simulink model "DCMG_SG"  (R2016a)
settings: Solver=FixedStepDiscrete  StartTime=0.0  StopTime=inf  FixedStep=.1  RelTol=1e-3
StartFcn:
  | h=add_exec_event_listener('GridSGHardware/GUIScope','PostOutputs',@GUIScope);
undefined symbols (not defined in the file or in its folder): Manual
libraries: opclib x4
settings Model: Creator=Don  LastModifiedBy=Microgrid_Project
settings DataIOCC: SaveFormat=Array  SignalLoggingSaveFormat=ModelDataLogs
settings OptimizationCC: ExpressionDepthLimit=2147483647
settings DebuggingCC: UnderspecifiedInitializationDetection=Classic  MergeDetectMultiDrivingBlocksExec=none  SolverPrmCheckMsg=warning  FcnCallInpInsideContextMsg=UseLocalSettings  StateNameClashWarn=warning
settings HardwareCC: ProdBitPerPointer=32  ProdLargestAtomicFloat=None  ProdIntDivRoundTo=Undefined  ProdEndianess=Unspecified  ProdWordSize=32  ProdHWDeviceType=32-bit Generic
settings ModelReferenceCC: PropagateSignalLabelsOutOfModel=off
settings GRTTargetCC: CombineOutputUpdateFcns=off  GRTInterface=on
settings ConfigComp: CovModelRefEnable=Off

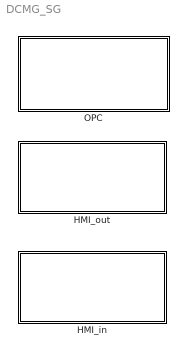
== system DCMG_SG ==
  HMI_in : Subsystem
  HMI_out : Subsystem
  OPC : Subsystem

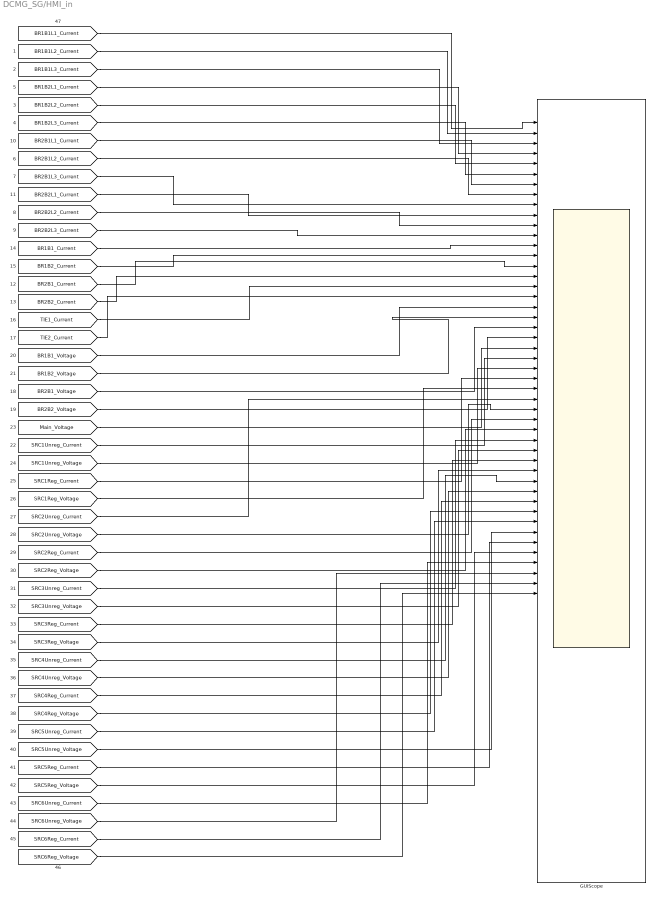
== system DCMG_SG/HMI_in ==
  GUIScope : Scope  NumInputPorts=73
  wires:
  [TIE2_Current] -> GUIScope/18
  [TIE1_Current] -> GUIScope/17
  [BR1B1_Voltage] -> GUIScope/19
  [BR2B2_Current] -> GUIScope/16
  [BR1B2_Voltage] -> GUIScope/20
  [BR2B1_Current] -> GUIScope/15
  [BR2B1_Voltage] -> GUIScope/21
  [BR1B2_Current] -> GUIScope/14
  [BR2B2_Voltage] -> GUIScope/22
  [BR1B1_Current] -> GUIScope/13
  [Main_Voltage] -> GUIScope/23
  [BR2B2L3_Current] -> GUIScope/12
  [SRC1Unreg_Current] -> GUIScope/24
  [BR2B2L2_Current] -> GUIScope/11
  [SRC1Unreg_Voltage] -> GUIScope/25
  [BR2B2L1_Current] -> GUIScope/10
  [SRC1Reg_Current] -> GUIScope/26
  [BR2B1L3_Current] -> GUIScope/9
  [SRC1Reg_Voltage] -> GUIScope/27
  [BR2B1L2_Current] -> GUIScope/8
  [SRC2Unreg_Current] -> GUIScope/28
  [BR2B1L1_Current] -> GUIScope/7
  [SRC2Unreg_Voltage] -> GUIScope/29
  [BR1B2L3_Current] -> GUIScope/6
  [SRC2Reg_Current] -> GUIScope/30
  [BR1B2L2_Current] -> GUIScope/5
  [SRC2Reg_Voltage] -> GUIScope/31
  [BR1B2L1_Current] -> GUIScope/4
  [SRC3Unreg_Current] -> GUIScope/32
  [BR1B1L3_Current] -> GUIScope/3
  [SRC3Unreg_Voltage] -> GUIScope/33
  [BR1B1L2_Current] -> GUIScope/2
  [SRC3Reg_Current] -> GUIScope/34
  [BR1B1L1_Current] -> GUIScope/1
  [SRC3Reg_Voltage] -> GUIScope/35
  [SRC4Unreg_Current] -> GUIScope/36
  [SRC4Unreg_Voltage] -> GUIScope/37
  [SRC4Reg_Current] -> GUIScope/38
  [SRC4Reg_Voltage] -> GUIScope/39
  [SRC5Unreg_Current] -> GUIScope/40
  [SRC5Unreg_Voltage] -> GUIScope/41
  [SRC5Reg_Current] -> GUIScope/42
  [SRC5Reg_Voltage] -> GUIScope/43
  [SRC6Unreg_Current] -> GUIScope/44
  [SRC6Unreg_Voltage] -> GUIScope/45
  [SRC6Reg_Current] -> GUIScope/46
  [SRC6Reg_Voltage] -> GUIScope/47

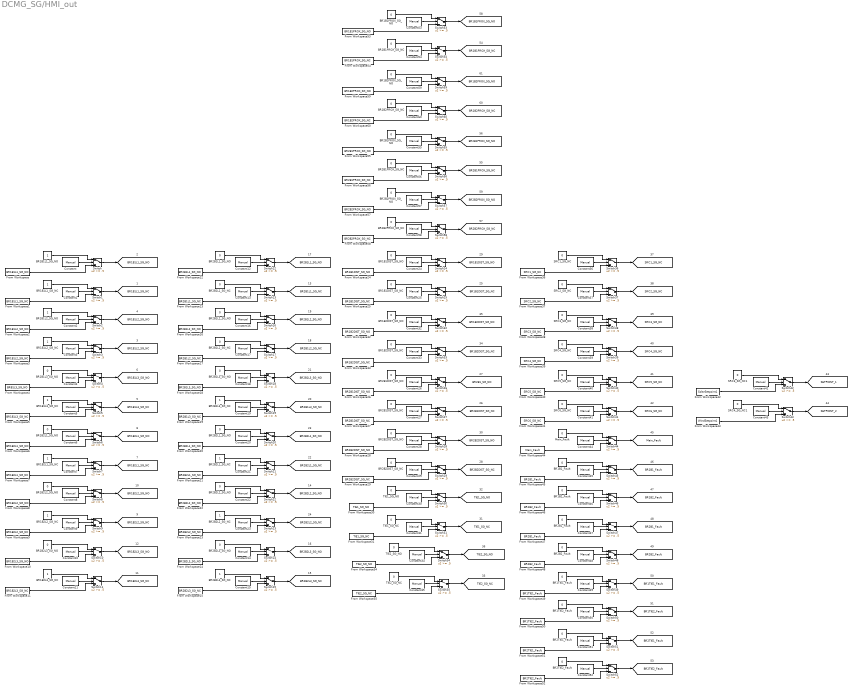
== system DCMG_SG/HMI_out ==
  BR1B1DIST_SG_NC : Constant  Value=0
  BR1B1DIST_SG_NO : Constant  Value=0
  BR1B1L1_SG_NC : Constant
  BR1B1L1_SG_NO : Constant
  BR1B1L2_SG_NC : Constant
  BR1B1L2_SG_NO : Constant
  BR1B1L3_SG_NC : Constant
  BR1B1L3_SG_NO : Constant  Value=0
  BR1B1PROX_SG_NC : Constant  Value=0
  BR1B1PROX_SG_NO : Constant  Value=0
  BR1B1_Fault : Constant  Value=0
  BR1B2DIST_SG_NC : Constant  Value=0
  BR1B2DIST_SG_NO : Constant  Value=0
  BR1B2L1_SG_NC : Constant
  BR1B2L1_SG_NO : Constant  Value=0
  BR1B2L2_SG_NC : Constant
  BR1B2L2_SG_NO : Constant  Value=0
  BR1B2L3_SG_NC : Constant
  BR1B2L3_SG_NO : Constant  Value=0
  BR1B2PROX_SG_NC : Constant  Value=0
  BR1B2PROX_SG_NO : Constant  Value=0
  BR1B2_Fault : Constant  Value=0
  BR1TIE1_Fault : Constant  Value=0
  BR1TIE2_Fault : Constant  Value=0
  BR2B1DIST_SG_NC : Constant  Value=0
  BR2B1DIST_SG_NO : Constant  Value=0
  BR2B1L1_SG_NC : Constant  Value=0
  BR2B1L1_SG_NO : Constant  Value=0
  BR2B1L2_SG_NC : Constant  Value=0
  BR2B1L2_SG_NO : Constant  Value=0
  BR2B1L3_SG_NC : Constant
  BR2B1L3_SG_NO : Constant  Value=0
  BR2B1PROX_SG_NC : Constant  Value=0
  BR2B1PROX_SG_NO : Constant  Value=0
  BR2B1_Fault : Constant  Value=0
  BR2B2DIST_SG_NC : Constant  Value=0
  BR2B2DIST_SG_NO : Constant  Value=0
  BR2B2L1_SG_NC : Constant
  BR2B2L1_SG_NO : Constant  Value=0
  BR2B2L2_SG_NC : Constant
  BR2B2L2_SG_NO : Constant  Value=0
  BR2B2L3_SG_NC : Constant
  BR2B2L3_SG_NO : Constant  Value=0
  BR2B2PROX_SG_NC : Constant  Value=0
  BR2B2PROX_SG_NO : Constant  Value=0
  BR2B2_Fault : Constant  Value=0
  BR2TIE1_Fault : Constant  Value=0
  BR2TIE2_Fault : Constant  Value=0
  Constant{,1..60} (61 alike) : Constant  Value=Manual
  From Workspace : FromWorkspace  VariableName=BR1B1L1_SG_NO  SampleTime=0  Interpolate=off  OutputAfterFinalValue=Holding final value
  From Workspace1 : FromWorkspace  VariableName=BR1B1L1_SG_NC  SampleTime=0  Interpolate=off  OutputAfterFinalValue=Holding final value
  From Workspace10 : FromWorkspace  VariableName=BR1B2L3_SG_NO  SampleTime=0  Interpolate=off  OutputAfterFinalValue=Holding final value
  From Workspace11 : FromWorkspace  VariableName=BR1B2L3_SG_NC  SampleTime=0  Interpolate=off  OutputAfterFinalValue=Holding final value
  From Workspace12 : FromWorkspace  VariableName=BR2B1L1_SG_NO  SampleTime=0  Interpolate=off  OutputAfterFinalValue=Holding final value
  From Workspace13 : FromWorkspace  VariableName=BR2B1L1_SG_NC  SampleTime=0  Interpolate=off  OutputAfterFinalValue=Holding final value
  From Workspace14 : FromWorkspace  VariableName=BR2B2L3_SG_NO  SampleTime=0  Interpolate=off  OutputAfterFinalValue=Holding final value
  From Workspace15 : FromWorkspace  VariableName=BR2B2L3_SG_NC  SampleTime=0  Interpolate=off  OutputAfterFinalValue=Holding final value
  From Workspace16 : FromWorkspace  VariableName=BR2B1L2_SG_NO  SampleTime=0  Interpolate=off  OutputAfterFinalValue=Holding final value
  From Workspace17 : FromWorkspace  VariableName=BR2B1L2_SG_NC  SampleTime=0  Interpolate=off  OutputAfterFinalValue=Holding final value
  From Workspace18 : FromWorkspace  VariableName=BR2B1L3_SG_NO  SampleTime=0  Interpolate=off  OutputAfterFinalValue=Holding final value
  From Workspace19 : FromWorkspace  VariableName=BR2B1L3_SG_NC  SampleTime=0  Interpolate=off  OutputAfterFinalValue=Holding final value
  From Workspace2 : FromWorkspace  VariableName=BR1B1L2_SG_NO  SampleTime=0  Interpolate=off  OutputAfterFinalValue=Holding final value
  From Workspace20 : FromWorkspace  VariableName=BR2B2L1_SG_NO  SampleTime=0  Interpolate=off  OutputAfterFinalValue=Holding final value
  From Workspace21 : FromWorkspace  VariableName=BR2B2L1_SG_NC  SampleTime=0  Interpolate=off  OutputAfterFinalValue=Holding final value
  From Workspace22 : FromWorkspace  VariableName=BR2B2L2_SG_NO  SampleTime=0  Interpolate=off  OutputAfterFinalValue=Holding final value
  From Workspace23 : FromWorkspace  VariableName=BR2B2L2_SG_NC  SampleTime=0  Interpolate=off  OutputAfterFinalValue=Holding final value
  From Workspace24 : FromWorkspace  VariableName=BR1B1DIST_SG_NO  SampleTime=0  Interpolate=off  OutputAfterFinalValue=Holding final value
  From Workspace25 : FromWorkspace  VariableName=BR1B1DIST_SG_NC  SampleTime=0  Interpolate=off  OutputAfterFinalValue=Holding final value
  From Workspace26 : FromWorkspace  VariableName=BR2B1DIST_SG_NO  SampleTime=0  Interpolate=off  OutputAfterFinalValue=Holding final value
  From Workspace27 : FromWorkspace  VariableName=BR2B1DIST_SG_NC  SampleTime=0  Interpolate=off  OutputAfterFinalValue=Holding final value
  From Workspace28 : FromWorkspace  VariableName=BR2B2DIST_SG_NO  SampleTime=0  Interpolate=off  OutputAfterFinalValue=Holding final value
  From Workspace29 : FromWorkspace  VariableName=BR2B2DIST_SG_NC  SampleTime=0  Interpolate=off  OutputAfterFinalValue=Holding final value
  From Workspace3 : FromWorkspace  VariableName=BR1B1L2_SG_NC  SampleTime=0  Interpolate=off  OutputAfterFinalValue=Holding final value
  From Workspace30 : FromWorkspace  VariableName=TIE1_SG_NO  SampleTime=0  Interpolate=off  OutputAfterFinalValue=Holding final value
  From Workspace31 : FromWorkspace  VariableName=TIE1_SG_NC  SampleTime=0  Interpolate=off  OutputAfterFinalValue=Holding final value
  From Workspace32 : FromWorkspace  VariableName=BR1B2DIST_SG_NO  SampleTime=0  Interpolate=off  OutputAfterFinalValue=Holding final value
  From Workspace33 : FromWorkspace  VariableName=BR1B2DIST_SG_NC  SampleTime=0  Interpolate=off  OutputAfterFinalValue=Holding final value
  From Workspace34 : FromWorkspace  VariableName=TIE2_SG_NO  SampleTime=0  Interpolate=off  OutputAfterFinalValue=Holding final value
  From Workspace35 : FromWorkspace  VariableName=TIE2_SG_NC  SampleTime=0  Interpolate=off  OutputAfterFinalValue=Holding final value
  From Workspace36 : FromWorkspace  VariableName=SRC1_SG_NC  SampleTime=0  Interpolate=off  OutputAfterFinalValue=Holding final value
  From Workspace37 : FromWorkspace  VariableName=SRC2_SG_NC  SampleTime=0  Interpolate=off  OutputAfterFinalValue=Holding final value
  From Workspace38 : FromWorkspace  VariableName=SRC3_SG_NC  SampleTime=0  Interpolate=off  OutputAfterFinalValue=Holding final value
  From Workspace39 : FromWorkspace  VariableName=SRC4_SG_NC  SampleTime=0  Interpolate=off  OutputAfterFinalValue=Holding final value
  From Workspace4 : FromWorkspace  VariableName=BRB1L3_SG_NO  SampleTime=0  Interpolate=off  OutputAfterFinalValue=Holding final value
  From Workspace40 : FromWorkspace  VariableName=SRC5_SG_NC  SampleTime=0  Interpolate=off  OutputAfterFinalValue=Holding final value
  From Workspace41 : FromWorkspace  VariableName=SRC6_SG_NC  SampleTime=0  Interpolate=off  OutputAfterFinalValue=Holding final value
  From Workspace42 : FromWorkspace  VariableName=SolarSetpoint1  SampleTime=0  Interpolate=off  OutputAfterFinalValue=Holding final value
  From Workspace43 : FromWorkspace  VariableName=WindSetpoint1  SampleTime=0  Interpolate=off  OutputAfterFinalValue=Holding final value
  From Workspace44 : FromWorkspace  VariableName=Main_Fault  SampleTime=0  Interpolate=off  OutputAfterFinalValue=Holding final value
  From Workspace45 : FromWorkspace  VariableName=BR1B1_Fault  SampleTime=0  Interpolate=off  OutputAfterFinalValue=Holding final value
  From Workspace46 : FromWorkspace  VariableName=BR1B2_Fault  SampleTime=0  Interpolate=off  OutputAfterFinalValue=Holding final value
  From Workspace47 : FromWorkspace  VariableName=BR2B1_Fault  SampleTime=0  Interpolate=off  OutputAfterFinalValue=Holding final value
  From Workspace48 : FromWorkspace  VariableName=BR2B2_Fault  SampleTime=0  Interpolate=off  OutputAfterFinalValue=Holding final value
  From Workspace49 : FromWorkspace  VariableName=BR1TIE1_Fault  SampleTime=0  Interpolate=off  OutputAfterFinalValue=Holding final value
  From Workspace5 : FromWorkspace  VariableName=BR1B1L3_SG_NC  SampleTime=0  Interpolate=off  OutputAfterFinalValue=Holding final value
  From Workspace50 : FromWorkspace  VariableName=BR1TIE2_Fault  SampleTime=0  Interpolate=off  OutputAfterFinalValue=Holding final value
  From Workspace51 : FromWorkspace  VariableName=BR2TIE1_Fault  SampleTime=0  Interpolate=off  OutputAfterFinalValue=Holding final value
  From Workspace52 : FromWorkspace  VariableName=BR2TIE2_Fault  SampleTime=0  Interpolate=off  OutputAfterFinalValue=Holding final value
  From Workspace53 : FromWorkspace  VariableName=BR1B1PROX_SG_NO  SampleTime=0  Interpolate=off  OutputAfterFinalValue=Holding final value
  From Workspace54 : FromWorkspace  VariableName=BR1B1PROX_SG_NC  SampleTime=0  Interpolate=off  OutputAfterFinalValue=Holding final value
  From Workspace55 : FromWorkspace  VariableName=BR2B1PROX_SG_NO  SampleTime=0  Interpolate=off  OutputAfterFinalValue=Holding final value
  From Workspace56 : FromWorkspace  VariableName=BR2B1PROX_SG_NC  SampleTime=0  Interpolate=off  OutputAfterFinalValue=Holding final value
  From Workspace57 : FromWorkspace  VariableName=BR2B2PROX_SG_NO  SampleTime=0  Interpolate=off  OutputAfterFinalValue=Holding final value
  From Workspace58 : FromWorkspace  VariableName=BR2B2PROX_SG_NC  SampleTime=0  Interpolate=off  OutputAfterFinalValue=Holding final value
  From Workspace59 : FromWorkspace  VariableName=BR1B2PROX_SG_NO  SampleTime=0  Interpolate=off  OutputAfterFinalValue=Holding final value
  From Workspace6 : FromWorkspace  VariableName=BR1B2L1_SG_NO  SampleTime=0  Interpolate=off  OutputAfterFinalValue=Holding final value
  From Workspace60 : FromWorkspace  VariableName=BR1B2PROX_SG_NC  SampleTime=0  Interpolate=off  OutputAfterFinalValue=Holding final value
  From Workspace7 : FromWorkspace  VariableName=BR1B2L1_SG_NC  SampleTime=0  Interpolate=off  OutputAfterFinalValue=Holding final value
  From Workspace8 : FromWorkspace  VariableName=BR1B2L2_SG_NO  SampleTime=0  Interpolate=off  OutputAfterFinalValue=Holding final value
  From Workspace9 : FromWorkspace  VariableName=BR1B2L2_SG_NC  SampleTime=0  Interpolate=off  OutputAfterFinalValue=Holding final value
  Main_Fault : Constant  Value=0
  SRC1_SG_NC : Constant  Value=0
  SRC2_SG_NC : Constant  Value=0
  SRC3_SG_NC : Constant  Value=0
  SRC3_SG_NC1 : Constant  Value=0
  SRC4_SG_NC : Constant  Value=0
  SRC4_SG_NC1 : Constant  Value=0
  SRC5_SG_NC : Constant  Value=0
  SRC6_SG_NC : Constant  Value=0
  Switch{,1..60} (61 alike) : Switch  Threshold=.5
  TIE1_SG_NC : Constant  Value=0
  TIE1_SG_NO : Constant  Value=0
  TIE2_SG_NC : Constant  Value=0
  TIE2_SG_NO : Constant  Value=0
  tag scope: BR1B1DIST_SG_NC=global, BR1B1DIST_SG_NO=global, BR1B1L1_SG_NC=global, BR1B1L1_SG_NO=global, BR1B1L2_SG_NC=global, BR1B1L2_SG_NO=global, BR1B1L3_SG_NC=global, BR1B1L3_SG_NO=global, BR1B1PROX_SG_NC=global, BR1B1PROX_SG_NO=global, BR1B1_Fault=global, BR1B2DIST_SG_NC=global, BR1B2DIST_SG_NO=global, BR1B2L1_SG_NC=global, BR1B2L1_SG_NO=global, BR1B2L2_SG_NC=global, BR1B2L2_SG_NO=global, BR1B2L3_SG_NC=global, BR1B2L3_SG_NO=global, BR1B2PROX_SG_NC=global, BR1B2PROX_SG_NO=global, BR1B2_Fault=global, BR1TIE1_Fault=global, BR1TIE2_Fault=global, BR2B1DIST_SG_NC=global, BR2B1L1_SG_NC=global, BR2B1L1_SG_NO=global, BR2B1L2_SG_NC=global, BR2B1L2_SG_NO=global, BR2B1L3_SG_NC=global, BR2B1L3_SG_NO=global, BR2B1PROX_SG_NC=global, BR2B1PROX_SG_NO=global, BR2B1_Fault=global, BR2B1_SG_NO=global, BR2B2DIST_SG_NC=global, BR2B2DIST_SG_NO=global, BR2B2L1_SG_NC=global, BR2B2L1_SG_NO=global, BR2B2L2_SG_NC=global, BR2B2L2_SG_NO=global, BR2B2L3_SG_NC=global, BR2B2L3_SG_NO=global, BR2B2PROX_SG_NC=global, BR2B2PROX_SG_NO=global, BR2B2_Fault=global, BR2TIE1_Fault=global, BR2TIE2_Fault=global, Main_Fault=global, SETPOINT_1=global, SETPOINT_2=global, SRC1_SG_NC=global, SRC2_SG_NC=global, SRC3_SG_NC=global, SRC4_SG_NC=global, SRC5_SG_NC=global, SRC6_SG_NC=global, TIE1_SG_NC=global, TIE1_SG_NO=global, TIE2_SG_NC=global, TIE2_SG_NO=global
  wires:
  Constant/1 -> Switch/2
  From Workspace/1 -> Switch/3
  BR1B1L1_SG_NO/1 -> Switch/1
  Switch/1 -> [BR1B1L1_SG_NO]
  Constant1/1 -> Switch1/2
  From Workspace1/1 -> Switch1/3
  BR1B1L1_SG_NC/1 -> Switch1/1
  Switch1/1 -> [BR1B1L1_SG_NC]
  Constant2/1 -> Switch2/2
  From Workspace2/1 -> Switch2/3
  BR1B1L2_SG_NO/1 -> Switch2/1
  Switch2/1 -> [BR1B1L2_SG_NO]
  Constant3/1 -> Switch3/2
  From Workspace3/1 -> Switch3/3
  BR1B1L2_SG_NC/1 -> Switch3/1
  Switch3/1 -> [BR1B1L2_SG_NC]
  Constant4/1 -> Switch4/2
  From Workspace4/1 -> Switch4/3
  BR1B1L3_SG_NO/1 -> Switch4/1
  Switch4/1 -> [BR1B1L3_SG_NO]
  Constant5/1 -> Switch5/2
  From Workspace5/1 -> Switch5/3
  BR1B1L3_SG_NC/1 -> Switch5/1
  Switch5/1 -> [BR1B1L3_SG_NC]
  Constant6/1 -> Switch6/2
  From Workspace6/1 -> Switch6/3
  BR1B2L1_SG_NO/1 -> Switch6/1
  Switch6/1 -> [BR1B2L1_SG_NO]
  Constant7/1 -> Switch7/2
  From Workspace7/1 -> Switch7/3
  BR1B2L1_SG_NC/1 -> Switch7/1
  Switch7/1 -> [BR1B2L1_SG_NC]
  Constant8/1 -> Switch8/2
  From Workspace8/1 -> Switch8/3
  BR1B2L2_SG_NO/1 -> Switch8/1
  Switch8/1 -> [BR1B2L2_SG_NO]
  Constant9/1 -> Switch9/2
  From Workspace9/1 -> Switch9/3
  BR1B2L2_SG_NC/1 -> Switch9/1
  Switch9/1 -> [BR1B2L2_SG_NC]
  Constant10/1 -> Switch10/2
  From Workspace10/1 -> Switch10/3
  BR1B2L3_SG_NO/1 -> Switch10/1
  Switch10/1 -> [BR1B2L3_SG_NO]
  Constant11/1 -> Switch11/2
  From Workspace11/1 -> Switch11/3
  BR1B2L3_SG_NC/1 -> Switch11/1
  Switch11/1 -> [BR1B2L3_SG_NC]
  Constant12/1 -> Switch12/2
  From Workspace12/1 -> Switch12/3
  BR2B1L1_SG_NO/1 -> Switch12/1
  Switch12/1 -> [BR2B1L1_SG_NO]
  Constant13/1 -> Switch13/2
  From Workspace13/1 -> Switch13/3
  BR2B1L1_SG_NC/1 -> Switch13/1
  Switch13/1 -> [BR2B1L1_SG_NC]
  Constant16/1 -> Switch16/2
  From Workspace16/1 -> Switch16/3
  BR2B1L2_SG_NO/1 -> Switch16/1
  Switch16/1 -> [BR2B1L2_SG_NO]
  Constant17/1 -> Switch17/2
  From Workspace17/1 -> Switch17/3
  BR2B1L2_SG_NC/1 -> Switch17/1
  Switch17/1 -> [BR2B1L2_SG_NC]
  Constant18/1 -> Switch18/2
  From Workspace18/1 -> Switch18/3
  BR2B1L3_SG_NO/1 -> Switch18/1
  Switch18/1 -> [BR2B1L3_SG_NO]
  Constant19/1 -> Switch19/2
  From Workspace19/1 -> Switch19/3
  BR2B1L3_SG_NC/1 -> Switch19/1
  Switch19/1 -> [BR2B1L3_SG_NC]
  Constant20/1 -> Switch20/2
  From Workspace20/1 -> Switch20/3
  BR2B2L1_SG_NO/1 -> Switch20/1
  Switch20/1 -> [BR2B2L1_SG_NO]
  Constant21/1 -> Switch21/2
  From Workspace21/1 -> Switch21/3
  BR2B2L1_SG_NC/1 -> Switch21/1
  Switch21/1 -> [BR2B2L1_SG_NC]
  Constant22/1 -> Switch22/2
  From Workspace22/1 -> Switch22/3
  BR2B2L2_SG_NO/1 -> Switch22/1
  Switch22/1 -> [BR2B2L2_SG_NO]
  Constant23/1 -> Switch23/2
  From Workspace23/1 -> Switch23/3
  BR2B2L2_SG_NC/1 -> Switch23/1
  Switch23/1 -> [BR2B2L2_SG_NC]
  Constant14/1 -> Switch14/2
  From Workspace14/1 -> Switch14/3
  BR2B2L3_SG_NO/1 -> Switch14/1
  Switch14/1 -> [BR2B2L3_SG_NO]
  Constant15/1 -> Switch15/2
  From Workspace15/1 -> Switch15/3
  BR2B2L3_SG_NC/1 -> Switch15/1
  Switch15/1 -> [BR2B2L3_SG_NC]
  Constant24/1 -> Switch24/2
  From Workspace24/1 -> Switch24/3
  BR1B1DIST_SG_NO/1 -> Switch24/1
  Switch24/1 -> [BR1B1DIST_SG_NO]
  Constant25/1 -> Switch25/2
  From Workspace25/1 -> Switch25/3
  BR1B1DIST_SG_NC/1 -> Switch25/1
  Switch25/1 -> [BR1B1DIST_SG_NC]
  Constant32/1 -> Switch32/2
  From Workspace32/1 -> Switch32/3
  BR1B2DIST_SG_NO/1 -> Switch32/1
  Switch32/1 -> [BR1B2DIST_SG_NO]
  Constant33/1 -> Switch33/2
  From Workspace33/1 -> Switch33/3
  BR1B2DIST_SG_NC/1 -> Switch33/1
  Switch33/1 -> [BR1B2DIST_SG_NC]
  Constant26/1 -> Switch26/2
  From Workspace26/1 -> Switch26/3
  BR2B1DIST_SG_NO/1 -> Switch26/1
  Switch26/1 -> [BR2B1_SG_NO]
  Constant27/1 -> Switch27/2
  From Workspace27/1 -> Switch27/3
  BR2B1DIST_SG_NC/1 -> Switch27/1
  Switch27/1 -> [BR2B1DIST_SG_NC]
  Constant28/1 -> Switch28/2
  From Workspace28/1 -> Switch28/3
  BR2B2DIST_SG_NO/1 -> Switch28/1
  Switch28/1 -> [BR2B2DIST_SG_NO]
  Constant29/1 -> Switch29/2
  From Workspace29/1 -> Switch29/3
  BR2B2DIST_SG_NC/1 -> Switch29/1
  Switch29/1 -> [BR2B2DIST_SG_NC]
  Constant30/1 -> Switch30/2
  From Workspace30/1 -> Switch30/3
  TIE1_SG_NO/1 -> Switch30/1
  Switch30/1 -> [TIE1_SG_NO]
  Constant31/1 -> Switch31/2
  From Workspace31/1 -> Switch31/3
  TIE1_SG_NC/1 -> Switch31/1
  Switch31/1 -> [TIE1_SG_NC]
  Constant34/1 -> Switch34/2
  From Workspace34/1 -> Switch34/3
  TIE2_SG_NO/1 -> Switch34/1
  Switch34/1 -> [TIE2_SG_NO]
  Constant35/1 -> Switch35/2
  From Workspace35/1 -> Switch35/3
  TIE2_SG_NC/1 -> Switch35/1
  Switch35/1 -> [TIE2_SG_NC]
  Constant36/1 -> Switch36/2
  From Workspace36/1 -> Switch36/3
  SRC1_SG_NC/1 -> Switch36/1
  Switch36/1 -> [SRC1_SG_NC]
  Constant37/1 -> Switch37/2
  From Workspace37/1 -> Switch37/3
  SRC2_SG_NC/1 -> Switch37/1
  Switch37/1 -> [SRC2_SG_NC]
  Constant38/1 -> Switch38/2
  From Workspace38/1 -> Switch38/3
  SRC3_SG_NC/1 -> Switch38/1
  Switch38/1 -> [SRC3_SG_NC]
  Constant39/1 -> Switch39/2
  From Workspace39/1 -> Switch39/3
  SRC4_SG_NC/1 -> Switch39/1
  Switch39/1 -> [SRC4_SG_NC]
  Constant40/1 -> Switch40/2
  From Workspace40/1 -> Switch40/3
  SRC5_SG_NC/1 -> Switch40/1
  Switch40/1 -> [SRC5_SG_NC]
  Constant41/1 -> Switch41/2
  From Workspace41/1 -> Switch41/3
  SRC6_SG_NC/1 -> Switch41/1
  Switch41/1 -> [SRC6_SG_NC]
  Constant42/1 -> Switch42/2
  From Workspace42/1 -> Switch42/3
  SRC3_SG_NC1/1 -> Switch42/1
  Switch42/1 -> [SETPOINT_1]
  Constant43/1 -> Switch43/2
  From Workspace43/1 -> Switch43/3
  SRC4_SG_NC1/1 -> Switch43/1
  Switch43/1 -> [SETPOINT_2]
  Constant44/1 -> Switch44/2
  From Workspace44/1 -> Switch44/3
  Main_Fault/1 -> Switch44/1
  Switch44/1 -> [Main_Fault]
  Constant45/1 -> Switch45/2
  From Workspace45/1 -> Switch45/3
  BR1B1_Fault/1 -> Switch45/1
  Switch45/1 -> [BR1B1_Fault]
  Constant46/1 -> Switch46/2
  From Workspace46/1 -> Switch46/3
  BR1B2_Fault/1 -> Switch46/1
  Switch46/1 -> [BR1B2_Fault]
  Constant47/1 -> Switch47/2
  From Workspace47/1 -> Switch47/3
  BR2B1_Fault/1 -> Switch47/1
  Switch47/1 -> [BR2B1_Fault]
  Constant48/1 -> Switch48/2
  From Workspace48/1 -> Switch48/3
  BR2B2_Fault/1 -> Switch48/1
  Switch48/1 -> [BR2B2_Fault]
  Constant49/1 -> Switch49/2
  From Workspace49/1 -> Switch49/3
  BR1TIE1_Fault/1 -> Switch49/1
  Switch49/1 -> [BR1TIE1_Fault]
  Constant50/1 -> Switch50/2
  From Workspace50/1 -> Switch50/3
  BR1TIE2_Fault/1 -> Switch50/1
  Switch50/1 -> [BR1TIE2_Fault]
  Constant51/1 -> Switch51/2
  From Workspace51/1 -> Switch51/3
  BR2TIE1_Fault/1 -> Switch51/1
  Switch51/1 -> [BR2TIE1_Fault]
  Constant52/1 -> Switch52/2
  From Workspace52/1 -> Switch52/3
  BR2TIE2_Fault/1 -> Switch52/1
  Switch52/1 -> [BR2TIE2_Fault]
  Constant53/1 -> Switch53/2
  From Workspace53/1 -> Switch53/3
  BR1B1PROX_SG_NO/1 -> Switch53/1
  Switch53/1 -> [BR1B1PROX_SG_NO]
  Constant54/1 -> Switch54/2
  From Workspace54/1 -> Switch54/3
  BR1B1PROX_SG_NC/1 -> Switch54/1
  Switch54/1 -> [BR1B1PROX_SG_NC]
  Constant59/1 -> Switch59/2
  From Workspace59/1 -> Switch59/3
  BR1B2PROX_SG_NO/1 -> Switch59/1
  Switch59/1 -> [BR1B2PROX_SG_NO]
  Constant60/1 -> Switch60/2
  From Workspace60/1 -> Switch60/3
  BR1B2PROX_SG_NC/1 -> Switch60/1
  Switch60/1 -> [BR1B2PROX_SG_NC]
  Constant55/1 -> Switch55/2
  From Workspace55/1 -> Switch55/3
  BR2B1PROX_SG_NO/1 -> Switch55/1
  Switch55/1 -> [BR2B1PROX_SG_NO]
  Constant56/1 -> Switch56/2
  From Workspace56/1 -> Switch56/3
  BR2B1PROX_SG_NC/1 -> Switch56/1
  Switch56/1 -> [BR2B1PROX_SG_NC]
  Constant57/1 -> Switch57/2
  From Workspace57/1 -> Switch57/3
  BR2B2PROX_SG_NO/1 -> Switch57/1
  Switch57/1 -> [BR2B2PROX_SG_NO]
  Constant58/1 -> Switch58/2
  From Workspace58/1 -> Switch58/3
  BR2B2PROX_SG_NC/1 -> Switch58/1
  Switch58/1 -> [BR2B2PROX_SG_NC]

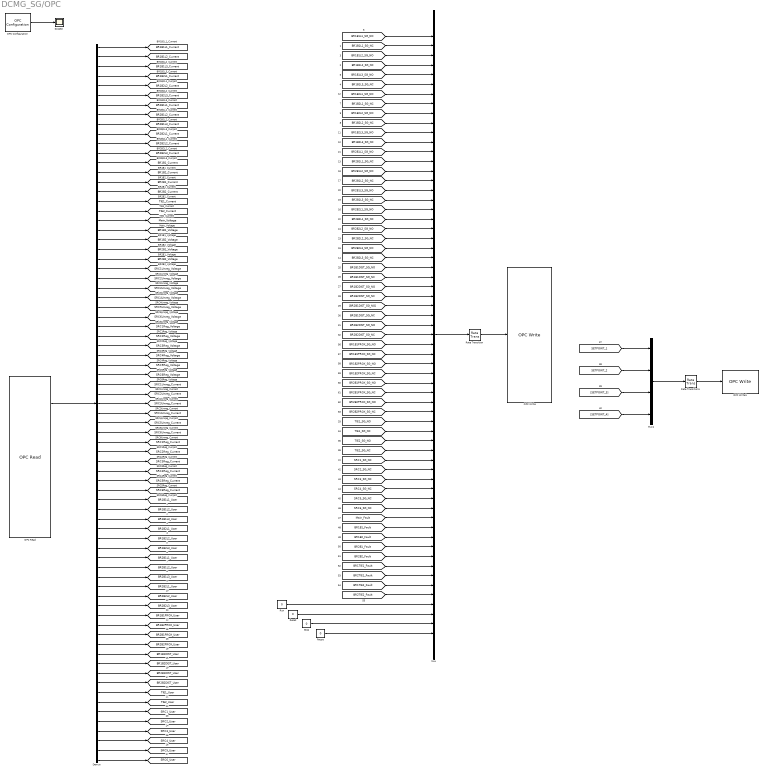
== system DCMG_SG/OPC ==
  Demux : Demux  Outputs=75
  Mux : Mux  Inputs=63
  Mux1 : Mux
  OPC Configuration : opclib/OPC Configuration  opcServers=localhost/FactoryTalk Gateway/10  errMissingItems=Error  errReadWrite=Warn  errShutdown=Error  errRTViolation=Warn  rtEnable=on  speedup=1  showLatency=on  beingUsed=on
  OPC Read : opclib/OPC Read  serverHost=localhost  serverID=FactoryTalk Gateway  itemIDs=::[smartgrid]Program:MainProgram.BRANCH_1_BUS_1_LOAD_1_Current, ::[smartgrid]Program:MainProgram.BRANCH_1_BUS_1_LOAD_2_Current, ::[smartgrid]Program:MainProgram.BRANCH_1_BUS_1_LOAD_3_Current, ::[smartgrid]Program:MainProgram.BRANCH_1_BUS_2_LOAD_1_Current, ::[smartgrid]Program:MainProgram.BRANCH_1_BUS_2_LOAD_2_Current, ::[smartgrid]Program:MainProgram.BRANCH_1_BUS_2_LOAD_3_Current, ::[smartgrid]Program:MainProgram.BRANCH_2_BUS_1_LOAD_1_Current, ::[smartgrid]Program:MainProgram.BRANCH_2_BUS_1_LOAD_2_Current, ::[smartgrid]Program:MainProgram.BRANCH_2_BUS_1_LOAD_3_Current, ::[smartgrid]Program:MainProgram.BRANCH_2_BUS_2_LOAD_1_Current, ::[smartgrid]Program:MainProgram.BRANCH_2_BUS_2_LOAD_2_Current, ::[smartgrid]Program:MainProgram.BRANCH_2_BUS_2_LOAD_3_Current, ::[smartgrid]Program:MainProgram.BRANCH_1_BUS_1_Current, ::[smartgrid]Program:MainProgram.BRANCH_1_BUS_2_Current, ::[smartgrid]Program:MainProgram.BRANCH_2_BUS_1_Current, ::[smartgrid]Program:MainProgram.BRANCH_2_BUS_2_Current, ::[smartgrid]Program:MainProgram.CROSSTIE_1_Current, ::[smartgrid]Program:MainProgram.CROSSTIE_2_Current, ::[smartgrid]Program:MainProgram.MAIN_BUS_Voltage, ::[smartgrid]Program:MainProgram.BRANCH_1_BUS_1_Voltage, ::[smartgrid]Program:MainProgram.BRANCH_1_BUS_2_Voltage, ::[smartgrid]Program:MainProgram.BRANCH_2_BUS_1_Voltage, ::[smartgrid]Program:MainProgram.BRANCH_2_BUS_2_Voltage, ::[smartgrid]Program:MainProgram.SOURCE_1_UnregVoltage, ::[smartgrid]Program:MainProgram.SOURCE_2_UnregVoltage, ::[smartgrid]Program:MainProgram.SOURCE_3_UnregVoltage, ::[smartgrid]Program:MainProgram.SOURCE_4_UnregVoltage, ::[smartgrid]Program:MainProgram.SOURCE_5_UnregVoltage, ::[smartgrid]Program:MainProgram.SOURCE_6_UnregVoltage, ::[smartgrid]Program:MainProgram.SOURCE_1_RegVoltage, ::[smartgrid]Program:MainProgram.SOURCE_2_RegVoltage, ::[smartgrid]Program:MainProgram.SOURCE_3_RegVoltage, ::[smartgrid]Program:MainProgram.SOURCE_4_RegVoltage, ::[smartgrid]Program:MainProgram.SOURCE_5_RegVoltage, ::[smartgrid]Program:MainProgram.SOURCE_6_RegVoltage, ::[smartgrid]Program:MainProgram.SOURCE_1_UnregCurrent, ::[smartgrid]Program:MainProgram.SOURCE_2_UnregCurrent, ::[smartgrid]Program:MainProgram.SOURCE_3_UnregCurrent, ::[smartgrid]Program:MainProgram.SOURCE_4_UnregCurrent, ::[smartgrid]Program:MainProgram.SOURCE_5_UnregCurrent, ::[smartgrid]Program:MainProgram.SOURCE_6_UnregCurrent, ::[smartgrid]Program:MainProgram.SOURCE_4_RegCurrent, ::[smartgrid]Program:MainProgram.SOURCE_5_RegCurrent, ::[smartgrid]Program:MainProgram.SOURCE_3_RegCurrent, ::[smartgrid]Program:MainProgram.SOURCE_1_RegCurrent, ::[smartgrid]Program:MainProgram.SOURCE_6_RegCurrent  readMode=Asynchronous (device)  dataType=double  updateRate=0.1  showQual=on  showTS=on  tsMode=Seconds since start
  OPC Write : opclib/OPC Write  serverHost=localhost  serverID=FactoryTalk Gateway  writeMode=Asynchronous  updateRate=0.1
  OPC Write1 : opclib/OPC Write  serverHost=localhost  serverID=FactoryTalk Gateway  itemIDs=[smartgrid]DCMicroGridreqStartup, [smartgrid]DCMicroGridreqShutdown, [smartgrid]DCMicroGridreqReset, [smartgrid]DCMicroGridisSimulating, [smartgrid]House01priority, [smartgrid]House02priority, [smartgrid]House03priority, [smartgrid]House04priority, [smartgrid]House05priority, [smartgrid]Load01priority, [smartgrid]Load02priority, [smartgrid]Load03priority, [smartgrid]Load04priority, [smartgrid]Load05priority, [smartgrid]Solar_Power, [smartgrid]SP_SG_Relay, [smartgrid]BG_SG_Relay, [smartgrid]RB_SG1_Relay, [smartgrid]RB_SG2_Relay, [smartgrid]RF_SG_Relay, [smartgrid]CB_SG1_Relay, [smartgrid]CB_SG2_Relay, [smartgrid]CF_SG_Relay, [smartgrid]RL1_SG1_Relay, [smartgrid]RL1_SG2_Relay, [smartgrid]RL2_SG1_Relay, [smartgrid]RL2_SG2_Relay, [smartgrid]RL3_SG1_Relay, [smartgrid]RL3_SG2_Relay, [smartgrid]RL4_SG1_Relay, [smartgrid]RL4_SG2_Relay, [smartgrid]RL5_SG1_Relay, [smartgrid]RL5_SG2_Relay, [smartgrid]CL1_SG1_Relay, [smartgrid]CL1_SG2_Relay, [smartgrid]CL2_SG1_Relay, [smartgrid]CL2_SG2_Relay, [smartgrid]CL3_SG1_Relay, [smartgrid]CL3_SG2_Relay, [smartgrid]CL4_SG1_Relay, [smartgrid]CL4_SG2_Relay, [smartgrid]CL5_SG1_Relay, [smartgrid]CL5_SG2_Relay  writeMode=Asynchronous  updateRate=0.1
  Pause : Constant  Value=0
  Rate Transition : RateTransition  OutPortSampleTime=.1
  Rate Transition1 : RateTransition  OutPortSampleTime=.1
  Reset : Constant  Value=0
  Run : Constant  Value=0
  Scope2 : Scope
  Stop : Constant  Value=0
  tag scope: BR1B1DIST_User=global, BR1B1L1_Current=global, BR1B1L1_User=global, BR1B1L2_Current=global, BR1B1L2_User=global, BR1B1L3_Current=global, BR1B1L3_User=global, BR1B1PROX_User=global, BR1B1_Current=global, BR1B1_Voltage=global, BR1B2DIST_User=global, BR1B2L1_Current=global, BR1B2L1_User=global, BR1B2L2_Current=global, BR1B2L2_User=global, BR1B2L3_Current=global, BR1B2L3_User=global, BR1B2PROX_User=global, BR1B2_Current=global, BR1B2_Voltage=global, BR2B1DIST_User=global, BR2B1L1_Current=global, BR2B1L1_User=global, BR2B1L2_Current=global, BR2B1L2_User=global, BR2B1L3_Current=global, BR2B1L3_User=global, BR2B1PROX_User=global, BR2B1_Current=global, BR2B1_Voltage=global, BR2B2DIST_User=global, BR2B2L1_Current=global, BR2B2L1_User=global, BR2B2L2_Current=global, BR2B2L2_User=global, BR2B2L3_Current=global, BR2B2L3_User=global, BR2B2PROX_User=global, BR2B2_Current=global, BR2B2_Voltage=global, Main_Voltage=global, SRC1Reg_Current=global, SRC1Reg_Voltage=global, SRC1Unreg_Current=global, SRC1Unreg_Voltage=global, SRC1_User=global, SRC2Reg_Current=global, SRC2Reg_Voltage=global, SRC2Unreg_Current=global, SRC2Unreg_Voltage=global, SRC2_User=global, SRC3Reg_Current=global, SRC3Reg_Voltage=global, SRC3Unreg_Current=global, SRC3Unreg_Voltage=global, SRC3_User=global, SRC4Reg_Current=global, SRC4Reg_Voltage=global, SRC4Unreg_Current=global, SRC4Unreg_Voltage=global, SRC4_User=global, SRC5Reg_Current=global, SRC5Reg_Voltage=global, SRC5Unreg_Current=global, SRC5Unreg_Voltage=global, SRC5_User=global, SRC6Reg_Current=global, SRC6Reg_Voltage=global, SRC6Unreg_Current=global, SRC6Unreg_Voltage=global, SRC6_User=global, TIE1_Current=global, TIE1_User=global, TIE2_Current=global, TIE2_User=global
  wires:
  OPC Configuration/1 -> Scope2/1
  OPC Read/1 -> Demux/1
  Mux/1 -> Rate Transition/1
  Rate Transition/1 -> OPC Write/1
  Demux/1 -> [BR1B1L1_Current]
  Demux/3 -> [BR1B1L3_Current]
  Demux/5 -> [BR1B2L2_Current]
  Demux/7 -> [BR2B1L1_Current]
  Demux/9 -> [BR2B1L3_Current]
  Demux/11 -> [BR2B2L2_Current]
  Demux/13 -> [BR1B1_Current]
  Demux/15 -> [BR2B1_Current]
  Demux/17 -> [TIE1_Current]
  Demux/19 -> [Main_Voltage]
  Demux/21 -> [BR1B2_Voltage]
  Demux/23 -> [BR2B2_Voltage]
  Demux/25 -> [SRC2Unreg_Voltage]
  Demux/27 -> [SRC4Unreg_Voltage]
  Demux/29 -> [SRC6Unreg_Voltage]
  Demux/31 -> [SRC2Reg_Voltage]
  Demux/33 -> [SRC4Reg_Voltage]
  Demux/35 -> [SRC6Reg_Voltage]
  Demux/37 -> [SRC2Unreg_Current]
  Demux/39 -> [SRC4Unreg_Current]
  Demux/41 -> [SRC6Unreg_Current]
  Demux/43 -> [SRC2Reg_Current]
  Demux/45 -> [SRC4Reg_Current]
  Demux/47 -> [SRC6Reg_Current]
  Demux/2 -> [BR1B1L2_Current]
  Demux/4 -> [BR1B2L1_Current]
  Demux/6 -> [BR1B2L3_Current]
  Demux/8 -> [BR2B1L2_Current]
  Demux/10 -> [BR2B2L1_Current]
  Demux/12 -> [BR2B2L3_Current]
  Demux/14 -> [BR1B2_Current]
  Demux/16 -> [BR2B2_Current]
  Demux/18 -> [TIE2_Current]
  Demux/20 -> [BR1B1_Voltage]
  Demux/22 -> [BR2B1_Voltage]
  Demux/24 -> [SRC1Unreg_Voltage]
  Demux/26 -> [SRC3Unreg_Voltage]
  Demux/28 -> [SRC5Unreg_Voltage]
  Demux/30 -> [SRC1Reg_Voltage]
  Demux/32 -> [SRC3Reg_Voltage]
  Demux/34 -> [SRC5Reg_Voltage]
  Demux/36 -> [SRC1Unreg_Current]
  Demux/38 -> [SRC3Unreg_Current]
  Demux/40 -> [SRC5Unreg_Current]
  Demux/42 -> [SRC1Reg_Current]
  Demux/44 -> [SRC3Reg_Current]
  Demux/46 -> [SRC5Reg_Current]
  [BR2B1L1_SG_NO] -> Mux/13
  [BR2B2DIST_SG_NO] -> Mux/31
  [BR1B2L3_SG_NC] -> Mux/12
  [BR1B2L2_SG_NO] -> Mux/9
  [BR1B1L1_SG_NO] -> Mux/1
  [BR2B2DIST_SG_NC] -> Mux/32
  [BR1B1L2_SG_NC] -> Mux/4
  [BR1B2L2_SG_NC] -> Mux/10
  [BR2B1L3_SG_NC] -> Mux/18
  [BR1B1L2_SG_NO] -> Mux/3
  [BR2B2L2_SG_NC] -> Mux/22
  [BR2B2L3_SG_NO] -> Mux/23
  [BR1B1L3_SG_NC] -> Mux/6
  [BR2B1L2_SG_NO] -> Mux/15
  [BR1B2DIST_SG_NO] -> Mux/27
  [BR1B1DIST_SG_NO] -> Mux/25
  [BR1B2L1_SG_NC] -> Mux/8
  [BR1B1L1_SG_NC] -> Mux/2
  [BR1B2L1_SG_NO] -> Mux/7
  [BR1B1L3_SG_NO] -> Mux/5
  [BR2B1DIST_SG_NO] -> Mux/29
  [BR2B1L2_SG_NC] -> Mux/16
  [BR2B2L3_SG_NC] -> Mux/24
  [BR2B1L1_SG_NC] -> Mux/14
  [BR2B2L1_SG_NC] -> Mux/20
  [BR2B2L1_SG_NO] -> Mux/19
  [BR1B2DIST_SG_NC] -> Mux/28
  [BR2B1L3_SG_NO] -> Mux/17
  [BR2B2L2_SG_NO] -> Mux/21
  [BR1B1DIST_SG_NC] -> Mux/26
  [BR2B1DIST_SG_NC] -> Mux/30
  [BR1B2L3_SG_NO] -> Mux/11
  Rate Transition1/1 -> OPC Write1/1
  [SETPOINT_2] -> Mux1/2
  [SETPOINT_4] -> Mux1/4
  [SETPOINT_3] -> Mux1/3
  [SETPOINT_1] -> Mux1/1
  Mux1/1 -> Rate Transition1/1
  [BR1B1PROX_SG_NO] -> Mux/33
  [BR2B1PROX_SG_NO] -> Mux/37
  [BR2B1PROX_SG_NC] -> Mux/38
  [BR1B2PROX_SG_NO] -> Mux/35
  [BR1B1PROX_SG_NC] -> Mux/34
  [BR2B2PROX_SG_NO] -> Mux/39
  [BR2B2PROX_SG_NC] -> Mux/40
  [BR1B2PROX_SG_NC] -> Mux/36
  [Main_Fault] -> Mux/51
  [TIE1_SG_NO] -> Mux/41
  [SRC4_SG_NC] -> Mux/48
  [SRC6_SG_NC] -> Mux/50
  [SRC2_SG_NC] -> Mux/46
  [TIE1_SG_NC] -> Mux/42
  [SRC5_SG_NC] -> Mux/49
  [BR1TIE2_Fault] -> Mux/58
  [SRC1_SG_NC] -> Mux/45
  [TIE2_SG_NO] -> Mux/43
  [BR1B2_Fault] -> Mux/53
  [TIE2_SG_NC] -> Mux/44
  [BR2B1_Fault] -> Mux/54
  [SRC3_SG_NC] -> Mux/47
  [BR1TIE1_Fault] -> Mux/56
  [BR2TIE2_Fault] -> Mux/59
  [BR2TIE1_Fault] -> Mux/57
  [BR1B1_Fault] -> Mux/52
  [BR2B2_Fault] -> Mux/55
  Pause/1 -> Mux/63
  Stop/1 -> Mux/62
  Reset/1 -> Mux/61
  Run/1 -> Mux/60
  Demux/48 -> [BR1B1L1_User]
  Demux/49 -> [BR1B1L2_User]
  Demux/50 -> [BR1B1L3_User]
  Demux/51 -> [BR1B2L1_User]
  Demux/52 -> [BR1B2L2_User]
  Demux/53 -> [BR1B2L3_User]
  Demux/54 -> [BR2B1L1_User]
  Demux/55 -> [BR2B1L2_User]
  Demux/56 -> [BR2B1L3_User]
  Demux/57 -> [BR2B2L1_User]
  Demux/58 -> [BR2B2L2_User]
  Demux/59 -> [BR2B2L3_User]
  Demux/60 -> [BR1B1PROX_User]
  Demux/61 -> [BR1B2PROX_User]
  Demux/62 -> [BR2B1PROX_User]
  Demux/63 -> [BR2B2PROX_User]
  Demux/64 -> [BR1B1DIST_User]
  Demux/65 -> [BR1B2DIST_User]
  Demux/66 -> [BR2B1DIST_User]
  Demux/67 -> [BR2B2DIST_User]
  Demux/68 -> [TIE1_User]
  Demux/69 -> [TIE2_User]
  Demux/70 -> [SRC1_User]
  Demux/71 -> [SRC2_User]
  Demux/72 -> [SRC3_User]
  Demux/73 -> [SRC4_User]
  Demux/74 -> [SRC5_User]
  Demux/75 -> [SRC6_User]
